simulink model "FlightControlSoftwareModules"  (R2024a)
settings: Solver=VariableStepAuto  StartTime=0.0  StopTime=50  RelTol=1e-3
PreLoadFcn:
  | load Data/PropData.mat;
  | F = 0;
InitFcn:
  | F = str2double(get_param('FlightControlSoftwareModules/Desired Velocity/Flight Phase','Value'));
undefined symbols (not defined in the file): PropData
libraries: slpidlib x1
settings Model: Creator=callie  LastModifiedBy=callie
settings DataIOCC: ReturnWorkspaceOutputs=off
settings DebuggingCC: AlgebraicLoopMsg=none

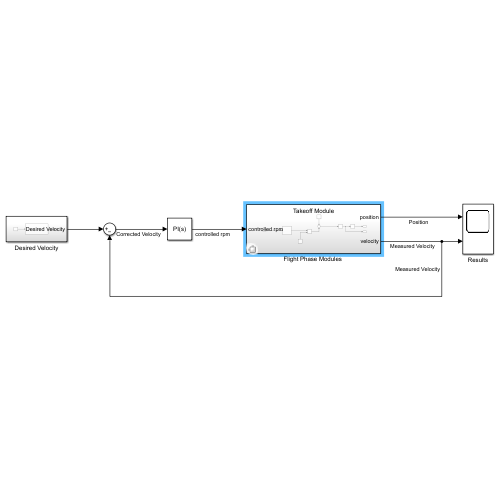
[thumbnail: Simulink's stored preview of the top-level diagram]
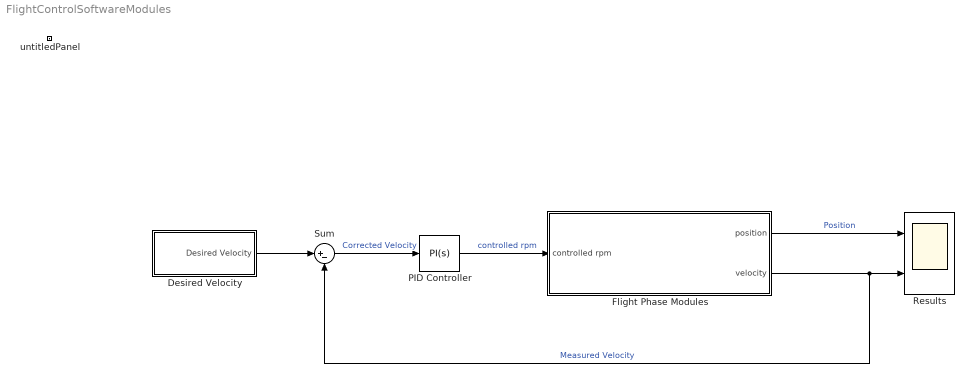
== system FlightControlSoftwareModules ==
  Desired Velocity : Subsystem
  "Flight Phase Modules " : Subsystem  Variant=on  AllowZeroVariantControls=on
  PID Controller : slpidlib/PID Controller  Controller=PI  Form=Parallel  TimeDomain=Continuous-time  UseExternalTs=off  SampleTime=-1  IntegratorMethod=Forward Euler  FilterMethod=Forward Euler  ControllerParametersSource=internal  P=28063.2903681465  I=4699.00310117393  UseKiTs=off  D=0  UseExternalDerivativeSource=off  N=100  UseFilter=on  TunerSelectOption=Transfer Function Based (PID Tuner App)  InitialConditionSource=internal  InitialConditionForIntegrator=0  InitialConditionForFilter=0  DifferentiatorICPrevScaledInput=0  ExternalReset=none  TrackingMode=off  Kt=1  LimitOutput=off  SatLimitsSource=internal  UpperSaturationLimit=inf  LowerSaturationLimit=-inf  LinearizeAsGain=on  AntiWindupMode=none  Kb=1  LimitIntegrator=off  UpperIntegratorSaturationLimit=inf  LowerIntegratorSaturationLimit=-inf  POutMin=[]  POutMax=[]  IOutMin=[]  IOutMax=[]  DOutMin=[]  DOutMax=[]  NOutMin=[]  NOutMax=[]  SumOutMin=[]  SumOutMax=[]  SaturationOutMin=[]  SaturationOutMax=[]  PParamMin=[]  PParamMax=[]  IParamMin=[]  IParamMax=[]  DParamMin=[]  DParamMax=[]  NParamMin=[]  NParamMax=[]  KbParamMin=[]  KbParamMax=[]  KtParamMin=[]  KtParamMax=[]  KbOutMin=[]  KbOutMax=[]  KtOutMin=[]  KtOutMax=[]  IntegratorOutMin=[]  IntegratorOutMax=[]  FilterOutMin=[]  FilterOutMax=[]  SumI1OutMin=[]  SumI1OutMax=[]  SumI2OutMin=[]  SumI2OutMax=[]  SumI3OutMin=[]  SumI3OutMax=[]  SumI4OutMin=[]  SumI4OutMax=[]  SumDOutMin=[]  SumDOutMax=[]  DifferentiatorOutMin=[]  DifferentiatorOutMax=[]  FilterDiffOutCoefMin=[]  FilterDiffOutCoefMax=[]  ReciprocalOutMin=[]  ReciprocalOutMax=[]  SumDenOutMin=[]  SumDenOutMax=[]  SumNumOutMin=[]  SumNumOutMax=[]  DivideOutMin=[]  DivideOutMax=[]  UdiffTsProdOutMin=[]  UdiffTsProdOutMax=[]  NTsProdOutMin=[]  NTsProdOutMax=[]  UintegralTsProdOutMin=[]  UintegralTsProdOutMax=[]  UngainTsProdOutMin=[]  UngainTsProdOutMax=[]  ClampingZeroOutDataTypeStr=Inherit: Inherit via back propagation  ClampingZeroOutMin=[]  ClampingZeroOutMax=[]  FilterDenConstantOutDataTypeStr=Inherit: Inherit via back propagation  FilterDenConstantOutMin=[]  FilterDenConstantOutMax=[]  PCopyOutDataTypeStr=Inherit: Inherit via back propagation  PCopyOutMin=[]  PCopyOutMax=[]  NCopyOutDataTypeStr=Inherit: Inherit via back propagation  NCopyOutMin=[]  NCopyOutMax=[]  IntegratorContinuousStateAttributes=''  IntegratorStateMustResolveToSignalObject=off  IntegratorRTWStateStorageClass=Auto  FilterContinuousStateAttributes=''  FilterStateMustResolveToSignalObject=off  FilterRTWStateStorageClass=Auto  ParallelPVariant=InternalParameters  IdealPVariant=Disabled  IVariant=InternalParameters  DVariant=Disabled  IntegratorVariant=Continuous  SatVariant=Disabled  AWVariant=Passthrough  PCopyVariant=Disabled  TRVariant=Disabled  FdbkBlocksVariant=Forward  IdealPFdbkVariant=Disabled  SatFdbkVariant=Disabled  DerivativeFilterVariant=Disabled  NVariant=Disabled  NCopyVariant=Disabled_SignalSpec  FilterICVariant=Disabled  IntegratorICVariant=InternalICs  ExternalResetVariant=Disabled  TRSumVariant=Passthrough  SumFdbkVariant=Disabled  SumVariant=Sum_PI  TsampFilterVariant=InternalTs  TsampNgainVariant=Passthrough  TsampIntegralVariant=Disabled_SignalSpec  ExternalSaturationOutDataTypeStr=Inherit: Same as second input  DerivativeSourceVariant=Disabled
  Results : Scope  NumInputPorts=2
  Sum : Sum  Inputs=|+-
  untitledPanel : Subsystem  Tag=HiddenForWebPanel  IsWebBlockPanel=on
  wires:
  PID Controller/1 -> "Flight Phase Modules "/1(controlled rpm)  "controlled rpm"
  "Flight Phase Modules "/1(position) -> Results/1  "Position"
  Sum/1 -> PID Controller/1  "Corrected Velocity"
  "Flight Phase Modules "/2(velocity) -> Sum/2, Results/2  "Measured Velocity"
  Desired Velocity/1(Desired Velocity) -> Sum/1

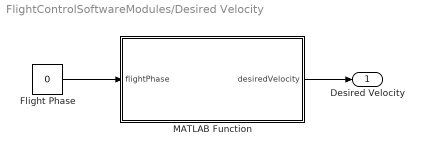
== system FlightControlSoftwareModules/Desired Velocity ==
  Flight Phase : Constant  Value=0
  MATLAB Function : MATLAB Function  TreatAsAtomicUnit=on
  Desired Velocity : Outport
  wires:
  Flight Phase/1 -> MATLAB Function/1(flightPhase)
  MATLAB Function/1(desiredVelocity) -> Desired Velocity/1

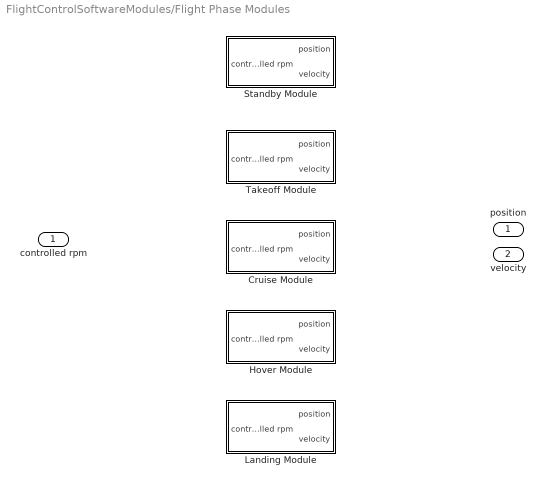
== system FlightControlSoftwareModules/Flight Phase Modules  ==
  controlled rpm : Inport
  Cruise Module : Subsystem  VariantControl=F == 2
  Hover Module : Subsystem  VariantControl=F == 3
  Landing Module : Subsystem  VariantControl=F == 4
  Standby Module : Subsystem  VariantControl=F == 0
  Takeoff Module : Subsystem  VariantControl=F == 1
  position : Outport
  velocity : Outport  Port=2

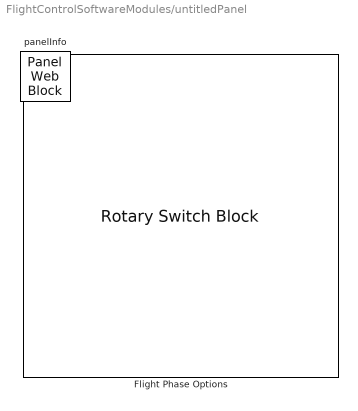
== system FlightControlSoftwareModules/untitledPanel ==
  Flight Phase Options : RotarySwitchBlock  Tag=HiddenForWebPanel  PanelInfo="{\"height\":226,\"left\":13,\"panelId\":\"panelId-ddc4f970-94dc-43de-9b9a-cf6499b59651\",\"top\":13,\"type\":\"panelChild\",\"version\":\"2019b\",\"width\":220,\"zIndex\":1500002}"  LabelPosition=Hide
      settings: Values={{'Standby', 'Takeoff', 'Cruise', 'Hover', 'Landing'}, [0 1 2 3 4]}
  panelInfo : PanelWebBlock  Tag=HiddenForWebPanel  PanelInfo="{\"compacted\":false,\"height\":252,\"isActiveTab\":true,\"left\":363,\"name\":\"Panel\",\"panelId\":\"panelId-ddc4f970-94dc-43de-9b9a-cf6499b59651\",\"popoutData\":{\"height\":0,\"left\":0,\"maximized\":false,\"top\":0,\"width\":0},\"popoutMode\":\"component\",\"tabIndex\":0,\"tabbedSetId\":\"tabbedSet2845638604\",\"top\":34,\"type\":\"panel\",\"version\":\"2019b\",\"visible\":true,\"width\":246,\"zIndex\":1500002}"  PanelSnapshot=<binary blob, 15872 chars, not shown>

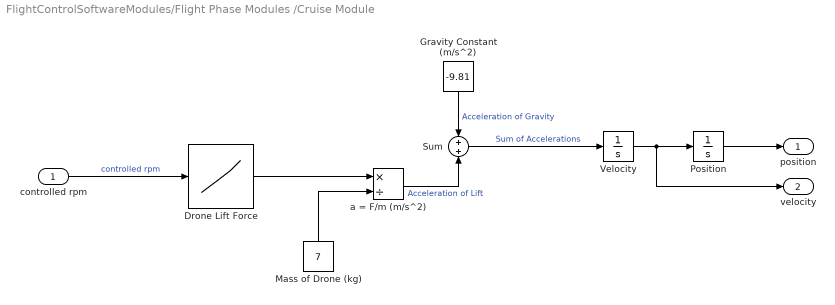
== system FlightControlSoftwareModules/Flight Phase Modules /Cruise Module ==
  controlled rpm : Inport
  Drone Lift Force : Lookup_n-D  NumberOfTableDimensions=1  BreakpointsForDimension1=PropData.rpm  Table=PropData.lift  InternalRulePriority=Speed  RndMeth=Simplest
  Gravity Constant (m/s^2) : Constant  Value=-9.81
  Mass of Drone (kg) : Constant  Value=7
  Position : Integrator  InitialCondition=77.9  LimitOutput=on  UpperSaturationLimit=77.9
  Sum : Sum  Inputs=+|+
  Velocity : Integrator
  a = F/m (m/s^2) : Product  Inputs=*/
  position : Outport
  velocity : Outport  Port=2
  wires:
  Mass of Drone (kg)/1 -> a = F/m (m/s^2)/2
  Velocity/1 -> velocity/1, Position/1
  Sum/1 -> Velocity/1  "Sum of Accelerations"
  Drone Lift Force/1 -> a = F/m (m/s^2)/1
  controlled rpm/1 -> Drone Lift Force/1  "controlled rpm"
  Position/1 -> position/1
  Gravity Constant (m/s^2)/1 -> Sum/1  "Acceleration of Gravity"
  a = F/m (m/s^2)/1 -> Sum/2  "Acceleration of Lift"

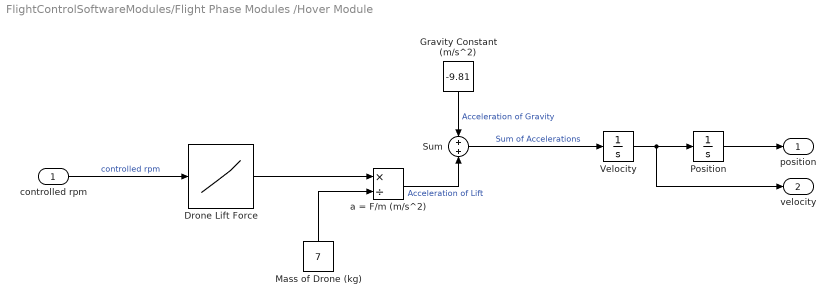
== system FlightControlSoftwareModules/Flight Phase Modules /Hover Module ==
  controlled rpm : Inport
  Drone Lift Force : Lookup_n-D  NumberOfTableDimensions=1  BreakpointsForDimension1=PropData.rpm  Table=PropData.lift*0.15  InternalRulePriority=Speed  RndMeth=Simplest
  Gravity Constant (m/s^2) : Constant  Value=-9.81
  Mass of Drone (kg) : Constant  Value=7
  Position : Integrator  InitialCondition=77.9
  Sum : Sum  Inputs=+|+
  Velocity : Integrator
  a = F/m (m/s^2) : Product  Inputs=*/
  position : Outport
  velocity : Outport  Port=2
  wires:
  Velocity/1 -> velocity/1, Position/1
  Drone Lift Force/1 -> a = F/m (m/s^2)/1
  Position/1 -> position/1
  a = F/m (m/s^2)/1 -> Sum/2  "Acceleration of Lift"
  Mass of Drone (kg)/1 -> a = F/m (m/s^2)/2
  controlled rpm/1 -> Drone Lift Force/1  "controlled rpm"
  Gravity Constant (m/s^2)/1 -> Sum/1  "Acceleration of Gravity"
  Sum/1 -> Velocity/1  "Sum of Accelerations"

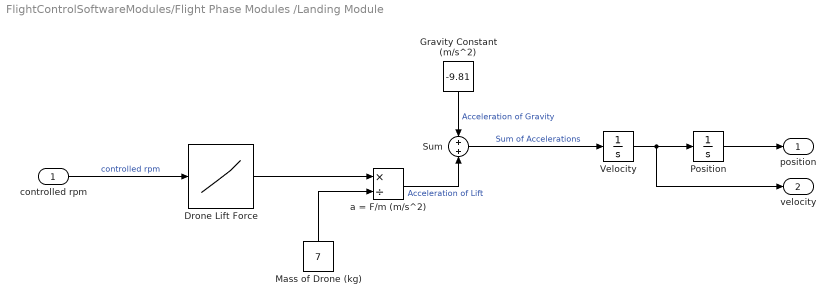
== system FlightControlSoftwareModules/Flight Phase Modules /Landing Module ==
  controlled rpm : Inport
  Drone Lift Force : Lookup_n-D  NumberOfTableDimensions=1  BreakpointsForDimension1=PropData.rpm  Table=PropData.lift*0.4  InternalRulePriority=Speed  RndMeth=Simplest
  Gravity Constant (m/s^2) : Constant  Value=-9.81
  Mass of Drone (kg) : Constant  Value=7
  Position : Integrator  InitialCondition=21.876  LowerSaturationLimit=0
  Sum : Sum  Inputs=+|+
  Velocity : Integrator
  a = F/m (m/s^2) : Product  Inputs=*/
  position : Outport
  velocity : Outport  Port=2
  wires:
  Mass of Drone (kg)/1 -> a = F/m (m/s^2)/2
  Velocity/1 -> velocity/1, Position/1
  Sum/1 -> Velocity/1  "Sum of Accelerations"
  Drone Lift Force/1 -> a = F/m (m/s^2)/1
  controlled rpm/1 -> Drone Lift Force/1  "controlled rpm"
  Position/1 -> position/1
  Gravity Constant (m/s^2)/1 -> Sum/1  "Acceleration of Gravity"
  a = F/m (m/s^2)/1 -> Sum/2  "Acceleration of Lift"

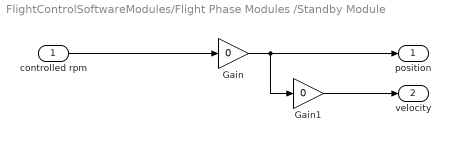
== system FlightControlSoftwareModules/Flight Phase Modules /Standby Module ==
  controlled rpm : Inport
  Gain : Gain  Gain=0
  Gain1 : Gain  Gain=0
  position : Outport
  velocity : Outport  Port=2
  wires:
  controlled rpm/1 -> Gain/1
  Gain/1 -> Gain1/1, position/1
  Gain1/1 -> velocity/1

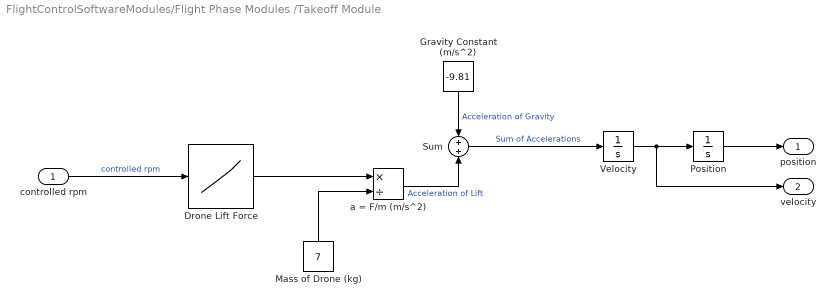
== system FlightControlSoftwareModules/Flight Phase Modules /Takeoff Module ==
  controlled rpm : Inport
  Drone Lift Force : Lookup_n-D  NumberOfTableDimensions=1  BreakpointsForDimension1=PropData.rpm  Table=PropData.lift  InternalRulePriority=Speed  RndMeth=Simplest
  Gravity Constant (m/s^2) : Constant  Value=-9.81
  Mass of Drone (kg) : Constant  Value=7
  Position : Integrator
  Sum : Sum  Inputs=+|+
  Velocity : Integrator
  a = F/m (m/s^2) : Product  Inputs=*/
  position : Outport
  velocity : Outport  Port=2
  wires:
  Mass of Drone (kg)/1 -> a = F/m (m/s^2)/2
  Velocity/1 -> velocity/1, Position/1
  Sum/1 -> Velocity/1  "Sum of Accelerations"
  Drone Lift Force/1 -> a = F/m (m/s^2)/1
  controlled rpm/1 -> Drone Lift Force/1  "controlled rpm"
  Position/1 -> position/1
  Gravity Constant (m/s^2)/1 -> Sum/1  "Acceleration of Gravity"
  a = F/m (m/s^2)/1 -> Sum/2  "Acceleration of Lift"

== matlab function FlightControlSoftwareModules/Desired Velocity/MATLAB Function ==
  data: flightPhase input; desiredVelocity output
function desiredVelocity  = velfcn(flightPhase)

if flightPhase == 1 % Takeoff
 desiredVelocity = 1.75;
elseif flightPhase == 2 % Cruise
 desiredVelocity = 10;
elseif flightPhase == 3 % Hover
 desiredVelocity = 0;
elseif flightPhase == 4 % Landing
 desiredVelocity = 0;
else % flightPhase == 0 % Standby
 desiredVelocity = 0;
end
